simulink model "mw_window"  (R2020a)
settings: Solver=VariableStepAuto  StartTime=0.0  StopTime=inf  RelTol=1e-3
InitFcn:
  | fs = 256e6;
libraries: hdlsllib x6, dspsigops x4, simulink x3
settings Model: Creator=david  LastModifiedBy=david
settings OptimizationCC: BlockReduction=off  ConditionallyExecuteInputs=off  DefaultParameterBehavior=Inlined
settings DebuggingCC: AlgebraicLoopMsg=error
settings HardwareCC: ProdBitPerPointer=32  ProdBitPerSizeT=32  ProdBitPerPtrDiffT=32  ProdLargestAtomicFloat=None  ProdIntDivRoundTo=Undefined  ProdEndianess=Unspecified  ProdWordSize=32  ProdHWDeviceType=ASIC/FPGA->ASIC/FPGA  TargetBitPerPointer=64  TargetBitPerSizeT=64  TargetBitPerPtrDiffT=64  TargetLongLongMode=on  TargetIntDivRoundTo=Zero  TargetEndianess=LittleEndian  TargetWordSize=64  TargetHWDeviceType=Custom Processor->MATLAB Host Computer  ProdEqTarget=off

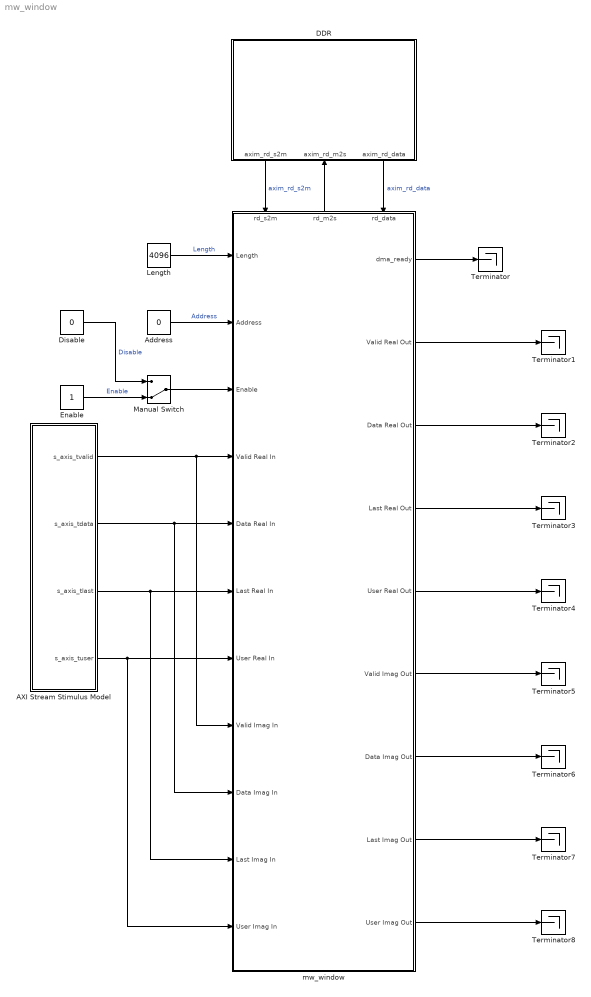
== system mw_window ==
  AXI Stream Stimulus Model : Subsystem
  Address : Constant  Value=0  OutDataTypeStr=uint32  SampleTime=1/fs
  DDR : Subsystem
      settings: PortSchema="{\"entries\":[{\"content\":{\"sides\":[{\"content\":{\"connectorIds\":[]},\"type\":\"ConnectorPlacement.EquallySpacedRectSide\",\"uuid\":\"2b557e1e-8026-43d3-80e6-d6d80e534d60\"},{\"content\":{\"connectorIds\":[\"Out1\",\"In1\",\"Out2\"],\"side\":\"RIGHT\"},\"type\":\"ConnectorPlacement.EquallySpacedRectSide\",\"uuid\":\"d37ff7b5-bcab-46eb-bf2f-7b890d421095\"},{\"content\":{\"connectorIds\":[],\"side\":\"TOP\"},\"type\":\"ConnectorPlacement.EquallySpacedRectSide\",\"uuid\":\"b7392330-958c-44c2-9b9d-e2e6efc00005\"}]},\"type\":\"ConnectorPlacement.EquallySpacedConnector\",\"uuid\":\"d6fedbd7-9a1a-42de-85f8-78943e8230da\"}],\"packageUris\":[\"http://schema.mathworks.com/mf0/Connector/19700101\"],\"version\":\"1.0\"}"
  Disable : Constant  Value=0  OutDataTypeStr=uint32  SampleTime=1/fs
  Enable : Constant  OutDataTypeStr=uint32  SampleTime=1/fs
  Length : Constant  Value=4096  OutDataTypeStr=uint32  SampleTime=1/fs
  Manual Switch : ManualSwitch  CurrentSetting=0
  Terminator{,1..8} (9 alike) : Terminator
  mw_window : Subsystem  TreatAsAtomicUnit=on
      settings: PortSchema="{\"entries\":[{\"content\":{\"sides\":[{\"content\":{\"connectorIds\":[\"In1\",\"In2\",\"In3\",\"In4\",\"In5\",\"In6\",\"In7\",\"In8\",\"In9\",\"In10\",\"In11\"]},\"type\":\"ConnectorPlacement.EquallySpacedRectSide\",\"uuid\":\"9bfde1a4-8e55-439d-ba95-b13ed8c2de82\"},{\"content\":{\"connectorIds\":[\"Out1\",\"Out2\",\"Out3\",\"Out4\",\"Out5\",\"Out6\",\"Out7\",\"Out8\",\"Out9\"],\"side\":\"RIGHT\"},\"type\":\"ConnectorPlacement.EquallySpacedRectSide\",\"uuid\":\"1fa858a7-8a79-448a-a9b9-a47438828a70\"},{\"content\":{\"connectorIds\":[\"In12\",\"Out10\",\"In13\"],\"side\":\"TOP\"},\"type\":\"ConnectorPlacement.EquallySpacedRectSide\",\"uuid\":\"fd991a14-ef2b-4cda-89a6-d580b9713fc0\"}]},\"type\":\"ConnectorPlacement.EquallySpacedConnector\",\"uuid\":\"ee399c2e-0a65-41c3-b55b-7131892126e8\"}],\"packageUris\":[\"http://schema.mathworks.com/mf0/Connector/19700101\"],\"version\":\"1.0\"}"
  wires:
  Length/1 -> mw_window/1(Length)  "Length"
  Address/1 -> mw_window/2(Address)  "Address"
  AXI Stream Stimulus Model/1(s_axis_tvalid) -> mw_window/8(Valid Imag In), mw_window/4(Valid Real In)
  AXI Stream Stimulus Model/2(s_axis_tdata) -> mw_window/9(Data Imag In), mw_window/5(Data Real In)
  AXI Stream Stimulus Model/4(s_axis_tuser) -> mw_window/7(User Real In), mw_window/11(User Imag In)
  AXI Stream Stimulus Model/3(s_axis_tlast) -> mw_window/10(Last Imag In), mw_window/6(Last Real In)
  DDR/2(axim_rd_s2m) -> mw_window/12(rd_s2m)  "axim_rd_s2m"
  mw_window/10(rd_m2s) -> DDR/1(axim_rd_m2s)
  DDR/1(axim_rd_data) -> mw_window/13(rd_data)  "axim_rd_data"
  mw_window/1(dma_ready) -> Terminator/1
  mw_window/2(Valid Real Out) -> Terminator1/1
  mw_window/3(Data Real Out) -> Terminator2/1
  mw_window/4(Last Real Out) -> Terminator3/1
  mw_window/5(User Real Out) -> Terminator4/1
  mw_window/6(Valid Imag Out) -> Terminator5/1
  mw_window/7(Data Imag Out) -> Terminator6/1
  mw_window/8(Last Imag Out) -> Terminator7/1
  mw_window/9(User Imag Out) -> Terminator8/1
  Manual Switch/1 -> mw_window/3(Enable)
  Disable/1 -> Manual Switch/1  "Disable"
  Enable/1 -> Manual Switch/2  "Enable"

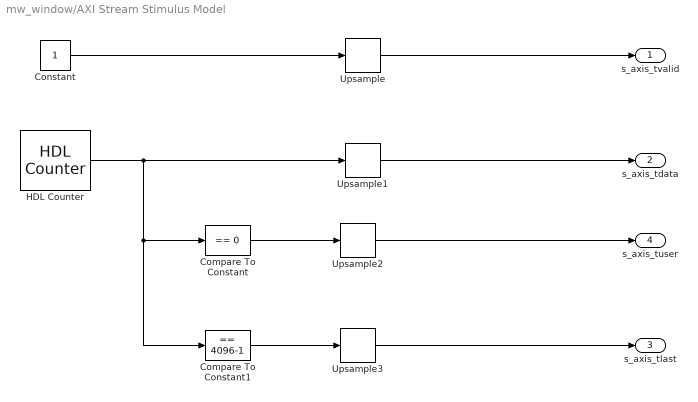
== system mw_window/AXI Stream Stimulus Model ==
  Compare To Constant : simulink/Logic and Bit Operations/Compare To Constant  relop===  const=0  OutDataTypeStr=boolean
  Compare To Constant1 : simulink/Logic and Bit Operations/Compare To Constant  relop===  const=4096-1  OutDataTypeStr=boolean
  Constant : Constant  OutDataTypeStr=boolean  SampleTime=-1
  HDL Counter : hdlsllib/Sources/HDL Counter  CountType=Count limited  CountInit=0  CountStep=1  CountMax=4096-1  CountFromType=Initial value  CountFrom=0  CountResetPort=off  CountLoadPort=off  CountEnbPort=off  CountDirPort=off  CountDataType=Unsigned  CountWordLen=16  CountFracLen=0  CountSampTime=-1
  Upsample{,1..3} (4 alike) : dspsigops/Upsample  N=2  phase=0  RateOptions=Allow multirate processing  ic=0  mode=Unused parameter value
  s_axis_tvalid : Outport
  s_axis_tdata : Outport  Port=2
  s_axis_tlast : Outport  Port=3
  s_axis_tuser : Outport  Port=4
  wires:
  Constant/1 -> Upsample/1
  Compare To Constant/1 -> Upsample2/1
  Compare To Constant1/1 -> Upsample3/1
  HDL Counter/1 -> Upsample1/1, Compare To Constant1/1, Compare To Constant/1
  Upsample/1 -> s_axis_tvalid/1
  Upsample1/1 -> s_axis_tdata/1
  Upsample2/1 -> s_axis_tuser/1
  Upsample3/1 -> s_axis_tlast/1

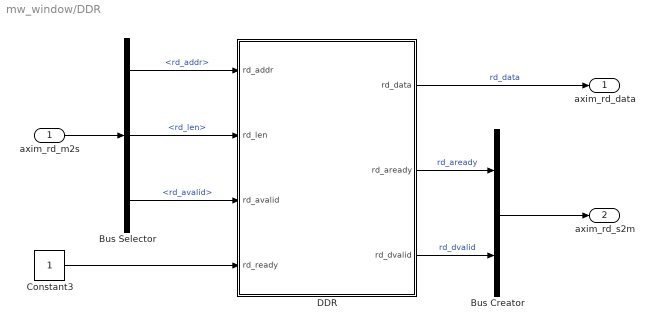
== system mw_window/DDR ==
  axim_rd_m2s : Inport
  Bus Creator : BusCreator  Inputs=2
  Bus Selector : BusSelector  OutputSignals=rd_addr,rd_len,rd_avalid
  Constant3 : Constant  OutDataTypeStr=boolean  SampleTime=-1
  DDR : Subsystem  mask{DDR_DATA=uint16(ones(1,4096)*2^15)}
      mask init:
      | %load('ram_data');
  axim_rd_data : Outport  VectorParamsAs1DForOutWhenUnconnected=off
  axim_rd_s2m : Outport  Port=2  VectorParamsAs1DForOutWhenUnconnected=off
  wires:
  Bus Creator/1 -> axim_rd_s2m/1
  DDR/1(rd_data) -> axim_rd_data/1  "rd_data"
  DDR/3(rd_dvalid) -> Bus Creator/2  "rd_dvalid"
  Constant3/1 -> DDR/4(rd_ready)
  Bus Selector/1 -> DDR/1(rd_addr)  "<rd_addr>"
  axim_rd_m2s/1 -> Bus Selector/1
  Bus Selector/3 -> DDR/3(rd_avalid)  "<rd_avalid>"
  DDR/2(rd_aready) -> Bus Creator/1  "rd_aready"
  Bus Selector/2 -> DDR/2(rd_len)  "<rd_len>"

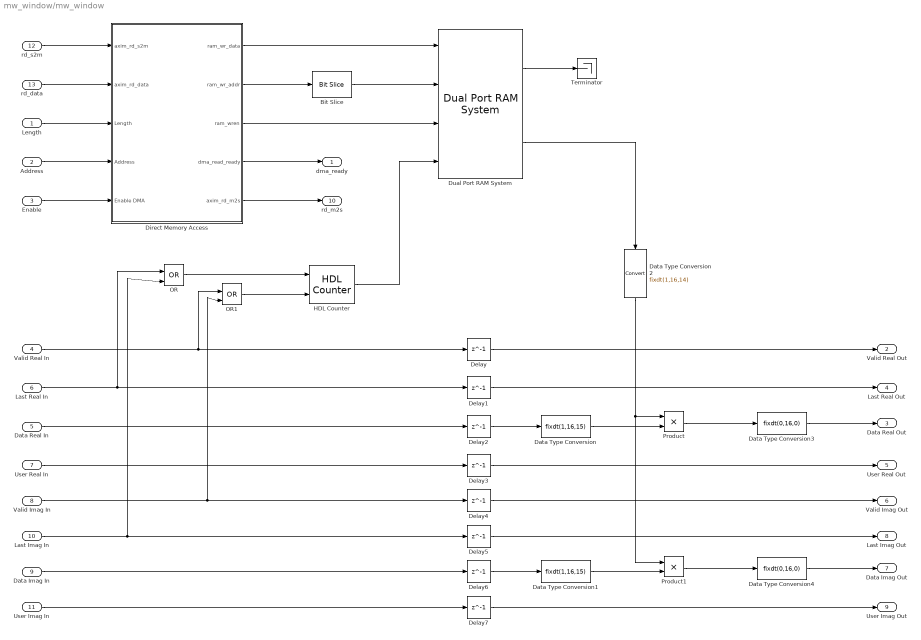
== system mw_window/mw_window ==
  Length : Inport
  Address : Inport  Port=2
  Enable : Inport  Port=3
  Valid Real In : Inport  Port=4
  Data Real In : Inport  Port=5
  Last Real In : Inport  Port=6
  User Real In : Inport  Port=7
  Valid Imag In : Inport  Port=8
  Data Imag In : Inport  Port=9
  Last Imag In : Inport  Port=10
  User Imag In : Inport  Port=11
  rd_s2m : Inport  Port=12
  rd_data : Inport  Port=13
  Bit Slice : hdlsllib/Logic and Bit Operations/Bit Slice  lidx=12  ridx=0
      settings: SourceProductBaseCode=SL
  Data Type Conversion : DataTypeConversion  OutDataTypeStr=fixdt(1,16,15)  ConvertRealWorld=Stored Integer (SI)
  Data Type Conversion1 : DataTypeConversion  OutDataTypeStr=fixdt(1,16,15)  ConvertRealWorld=Stored Integer (SI)
  Data Type Conversion2 : DataTypeConversion  OutDataTypeStr=fixdt(1,16,14)  ConvertRealWorld=Stored Integer (SI)
  Data Type Conversion3 : DataTypeConversion  OutDataTypeStr=fixdt(0,16,0)  ConvertRealWorld=Stored Integer (SI)
  Data Type Conversion4 : DataTypeConversion  OutDataTypeStr=fixdt(0,16,0)  ConvertRealWorld=Stored Integer (SI)
  Delay{,1..7} (8 alike) : Delay  DelayLength=1
  Direct Memory Access : Subsystem
  Dual Port RAM System : hdlsllib/HDL RAMs/Dual Port RAM System  RAMType=Dual port  WriteOutputValue=New data  RAMInitialValue=ones(1, 2^13)*2^14  SimulateUsing=Code generation
      settings: SourceProductBaseCode=SL
  HDL Counter : hdlsllib/Sources/HDL Counter  CountType=Count limited  CountInit=0  CountStep=1  CountMax=4095  CountFromType=Initial value  CountFrom=0  CountResetPort=on  CountLoadPort=off  CountEnbPort=on  CountDirPort=off  CountDataType=Unsigned  CountWordLen=13  CountFracLen=0  CountSampTime=1
  OR : Logic  Operator=OR  IconShape=distinctive  AllPortsSameDT=off  OutDataTypeStr=boolean
  OR1 : Logic  Operator=OR  IconShape=distinctive  AllPortsSameDT=off  OutDataTypeStr=boolean
  Product : Product  OutDataTypeStr=fixdt(1,16,15)  RndMeth=Round  SaturateOnIntegerOverflow=on
  Product1 : Product  OutDataTypeStr=fixdt(1,16,15)  RndMeth=Round  SaturateOnIntegerOverflow=on
  Terminator : Terminator
  dma_ready : Outport
  Valid Real Out : Outport  Port=2
  Data Real Out : Outport  Port=3
  Last Real Out : Outport  Port=4
  User Real Out : Outport  Port=5
  Valid Imag Out : Outport  Port=6
  Data Imag Out : Outport  Port=7
  Last Imag Out : Outport  Port=8
  User Imag Out : Outport  Port=9
  rd_m2s : Outport  Port=10
  wires:
  Address/1 -> Direct Memory Access/4(Address)
  Enable/1 -> Direct Memory Access/5(Enable DMA)
  Length/1 -> Direct Memory Access/3(Length)
  Direct Memory Access/1(ram_wr_data) -> Dual Port RAM System/1
  Direct Memory Access/2(ram_wr_addr) -> Bit Slice/1
  Direct Memory Access/3(ram_wren) -> Dual Port RAM System/3
  Direct Memory Access/4(dma_read_ready) -> dma_ready/1
  HDL Counter/1 -> Dual Port RAM System/4
  Valid Real In/1 -> OR1/1, Delay/1
  Last Real In/1 -> OR/1, Delay1/1
  Dual Port RAM System/1 -> Terminator/1
  Direct Memory Access/5(axim_rd_m2s) -> rd_m2s/1
  Dual Port RAM System/2 -> Data Type Conversion2/1
  Data Real In/1 -> Delay2/1
  Product/1 -> Data Type Conversion3/1
  User Real In/1 -> Delay3/1
  OR/1 -> HDL Counter/1
  OR1/1 -> HDL Counter/2
  Last Imag In/1 -> OR/2, Delay5/1
  Valid Imag In/1 -> OR1/2, Delay4/1
  Data Imag In/1 -> Delay6/1
  Product1/1 -> Data Type Conversion4/1
  User Imag In/1 -> Delay7/1
  rd_s2m/1 -> Direct Memory Access/1(axim_rd_s2m)
  rd_data/1 -> Direct Memory Access/2(axim_rd_data)
  Data Type Conversion/1 -> Product/2
  Data Type Conversion1/1 -> Product1/2
  Data Type Conversion2/1 -> Product1/1, Product/1
  Data Type Conversion3/1 -> Data Real Out/1
  Data Type Conversion4/1 -> Data Imag Out/1
  Delay/1 -> Valid Real Out/1
  Delay1/1 -> Last Real Out/1
  Delay2/1 -> Data Type Conversion/1
  Delay3/1 -> User Real Out/1
  Delay4/1 -> Valid Imag Out/1
  Delay5/1 -> Last Imag Out/1
  Delay6/1 -> Data Type Conversion1/1
  Delay7/1 -> User Imag Out/1
  Bit Slice/1 -> Dual Port RAM System/2

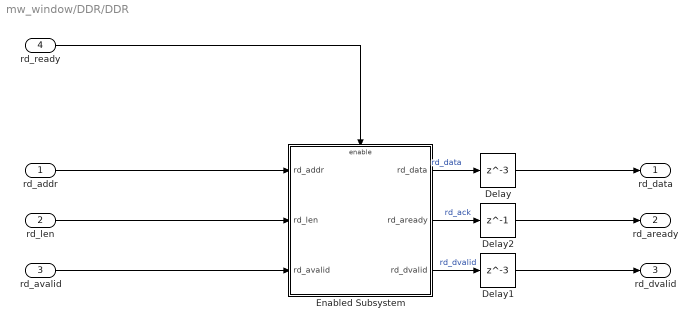
== system mw_window/DDR/DDR ==
  rd_addr : Inport
  rd_len : Inport  Port=2
  rd_avalid : Inport  Port=3
  rd_ready : Inport  Port=4
  Delay : Delay  DelayLength=3
  Delay1 : Delay  DelayLength=3
  Delay2 : Delay  DelayLength=1
  Enabled Subsystem : Subsystem  TreatAsAtomicUnit=on
  rd_data : Outport  VectorParamsAs1DForOutWhenUnconnected=off
  rd_aready : Outport  Port=2  VectorParamsAs1DForOutWhenUnconnected=off
  rd_dvalid : Outport  Port=3  VectorParamsAs1DForOutWhenUnconnected=off
  wires:
  Delay2/1 -> rd_aready/1
  Delay1/1 -> rd_dvalid/1
  Enabled Subsystem/3(rd_dvalid) -> Delay1/1  "rd_dvalid"
  rd_ready/1 -> Enabled Subsystem/Enable
  Enabled Subsystem/2(rd_aready) -> Delay2/1  "rd_ack"
  rd_avalid/1 -> Enabled Subsystem/3(rd_avalid)
  Delay/1 -> rd_data/1
  Enabled Subsystem/1(rd_data) -> Delay/1  "rd_data"
  rd_len/1 -> Enabled Subsystem/2(rd_len)
  rd_addr/1 -> Enabled Subsystem/1(rd_addr)

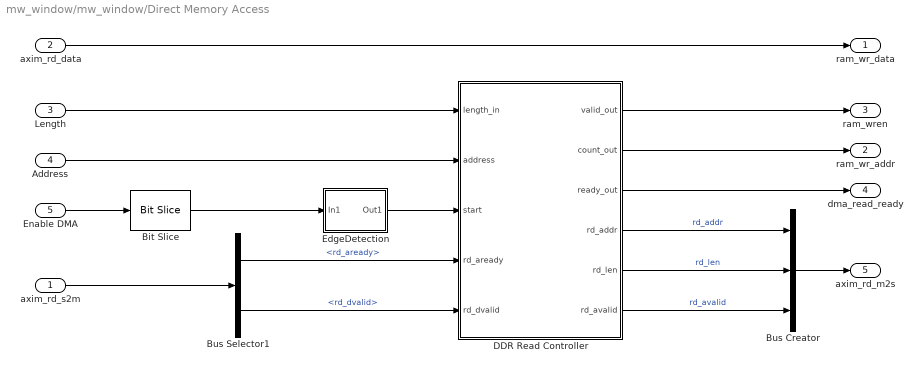
== system mw_window/mw_window/Direct Memory Access ==
  axim_rd_s2m : Inport
  axim_rd_data : Inport  Port=2
  Length : Inport  Port=3
  Address : Inport  Port=4
  Enable DMA : Inport  Port=5
  Bit Slice : hdlsllib/Logic and Bit Operations/Bit Slice  lidx=0  ridx=0
      settings: SourceProductBaseCode=SL
  Bus Creator : BusCreator  Inputs=3
  Bus Selector1 : BusSelector  OutputSignals=rd_aready,rd_dvalid
  DDR Read Controller : MATLAB Function  TreatAsAtomicUnit=on
  EdgeDetection : Subsystem
  ram_wr_data : Outport  VectorParamsAs1DForOutWhenUnconnected=off
  ram_wr_addr : Outport  Port=2  VectorParamsAs1DForOutWhenUnconnected=off
  ram_wren : Outport  Port=3  VectorParamsAs1DForOutWhenUnconnected=off
  dma_read_ready : Outport  Port=4  VectorParamsAs1DForOutWhenUnconnected=off
  axim_rd_m2s : Outport  Port=5  VectorParamsAs1DForOutWhenUnconnected=off
  wires:
  Enable DMA/1 -> Bit Slice/1
  Address/1 -> DDR Read Controller/2(address)
  DDR Read Controller/4(rd_addr) -> Bus Creator/1  "rd_addr"
  DDR Read Controller/6(rd_avalid) -> Bus Creator/3  "rd_avalid"
  Bus Creator/1 -> axim_rd_m2s/1
  DDR Read Controller/5(rd_len) -> Bus Creator/2  "rd_len"
  Bus Selector1/1 -> DDR Read Controller/4(rd_aready)  "<rd_aready>"
  axim_rd_s2m/1 -> Bus Selector1/1
  Bus Selector1/2 -> DDR Read Controller/5(rd_dvalid)  "<rd_dvalid>"
  axim_rd_data/1 -> ram_wr_data/1
  DDR Read Controller/2(count_out) -> ram_wr_addr/1
  DDR Read Controller/1(valid_out) -> ram_wren/1
  EdgeDetection/1(Out1) -> DDR Read Controller/3(start)
  DDR Read Controller/3(ready_out) -> dma_read_ready/1
  Length/1 -> DDR Read Controller/1(length_in)
  Bit Slice/1 -> EdgeDetection/1(In1)

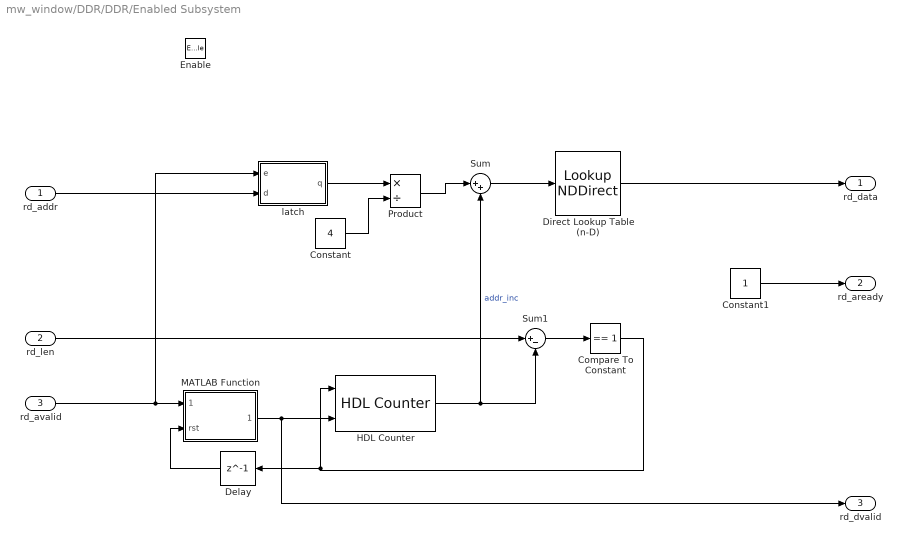
== system mw_window/DDR/DDR/Enabled Subsystem ==
  rd_addr : Inport
  rd_len : Inport  Port=2
  rd_avalid : Inport  Port=3
  Enable : EnablePort
  Compare To Constant : simulink/Logic and Bit Operations/Compare To Constant  relop===  const=1  OutDataTypeStr=boolean
  Constant : Constant  Value=4  SampleTime=-1
  Constant1 : Constant  OutDataTypeStr=boolean  SampleTime=-1
  Delay : Delay  DelayLength=1
  Direct Lookup Table (n-D) : LookupNDDirect  NumberOfTableDimensions=1  Table=DDR_DATA  DiagnosticForOutOfRangeInput=Error
  HDL Counter : hdlsllib/Sources/HDL Counter  CountType=Count limited  CountInit=0  CountStep=1  CountMax=2^16-1  CountFromType=Specify  CountFrom=0  CountResetPort=on  CountLoadPort=off  CountEnbPort=on  CountDirPort=off  CountDataType=Unsigned  CountWordLen=16  CountFracLen=0  CountSampTime=1
  MATLAB Function : MATLAB Function  TreatAsAtomicUnit=on
  Product : Product  Inputs=*/
  Sum : Sum  Inputs=|++  OutDataTypeStr=uint32
  Sum1 : Sum  Inputs=|+-
  latch : Subsystem
  rd_data : Outport  VectorParamsAs1DForOutWhenUnconnected=off
  rd_aready : Outport  Port=2  VectorParamsAs1DForOutWhenUnconnected=off
  rd_dvalid : Outport  Port=3  VectorParamsAs1DForOutWhenUnconnected=off
  wires:
  Constant1/1 -> rd_aready/1
  Delay/1 -> MATLAB Function/2(rst)
  Constant/1 -> Product/2
  Product/1 -> Sum/1
  latch/1(q) -> Product/1
  MATLAB Function/1(start_counter) -> HDL Counter/2, rd_dvalid/1
  rd_avalid/1 -> MATLAB Function/1(rd_avalid), latch/1(e)
  rd_len/1 -> Sum1/1
  rd_addr/1 -> latch/2(d)
  Compare To Constant/1 -> HDL Counter/1, Delay/1
  Sum/1 -> Direct Lookup Table (n-D)/1
  Sum1/1 -> Compare To Constant/1
  HDL Counter/1 -> Sum/2, Sum1/2  "addr_inc"
  Direct Lookup Table (n-D)/1 -> rd_data/1

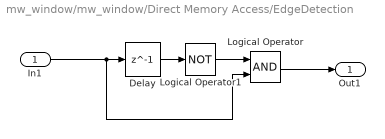
== system mw_window/mw_window/Direct Memory Access/EdgeDetection ==
  In1 : Inport
  Delay : Delay  DelayLength=1
  Logical Operator : Logic  AllPortsSameDT=off  OutDataTypeStr=boolean
  Logical Operator1 : Logic  Operator=NOT  AllPortsSameDT=off  OutDataTypeStr=boolean
  Out1 : Outport  VectorParamsAs1DForOutWhenUnconnected=off
  wires:
  Logical Operator/1 -> Out1/1
  Logical Operator1/1 -> Logical Operator/1
  Delay/1 -> Logical Operator1/1
  In1/1 -> Delay/1, Logical Operator/2

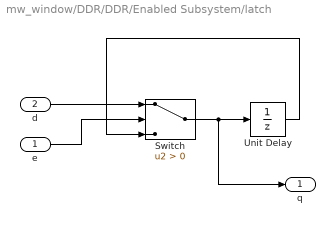
== system mw_window/DDR/DDR/Enabled Subsystem/latch ==
  e : Inport  OutDataTypeStr=boolean
  d : Inport  Port=2
  Switch : Switch  Criteria=u2 > Threshold
  Unit Delay : UnitDelay  SampleTime=-1  HasFrameUpgradeWarning=on
  q : Outport  VectorParamsAs1DForOutWhenUnconnected=off
  wires:
  Switch/1 -> Unit Delay/1, q/1
  e/1 -> Switch/2
  Unit Delay/1 -> Switch/3
  d/1 -> Switch/1

== matlab function mw_window/DDR/DDR/Enabled Subsystem/MATLAB Function ==
  data: rd_avalid input; start_counter output; rst input
function start_counter  = fcn(rd_avalid, rst)

persistent start;
if(isempty(start))
    start = false;
end

if (rd_avalid == true)
    start = true;
else
    
    if (rst == true)
        start = false;
    else
        start = start;
    end
end
start_counter = start;

== matlab function mw_window/Direct Memory Access/DDR Read Controller ==
  data: valid_out output boolean; count_out output; ready_out output boolean; length_in input; address input; start input boolean; rd_aready input; rd_dvalid input; rd_addr output uint32; rd_len output; rd_avalid output
function [valid_out,count_out,ready_out,rd_addr,rd_len,rd_avalid] = ddr_read_control(length_in, address, start, rd_aready, rd_dvalid)

% Create persistent variables (registers)
persistent burst_stop
if(isempty(burst_stop))
    burst_stop = uint16(0);
end
persistent burst_count;
if(isempty(burst_count))
    burst_count = uint16(0);
end
persistent rstate;
if isempty(rstate)
    rstate = fi(0, 0, 4, 0);
end


% State Memory Encoding
IDLE             = fi(1, 0, 4, 0);
READ_BURST_START = fi(2, 0, 4, 0);
DATA_COUNT       = fi(4, 0, 4, 0);

% Read control state machine
switch (rstate)
    case IDLE
        % output to AXI4 Master
        rd_addr = address;
        rd_len = uint16(0);
        rd_avalid = false;
        
        % output to DUT
        valid_out = false;
        ready_out = true;
        count_out = uint16(0);
        
        % State vars
        burst_count = uint16(0);
        burst_stop = uint16(length_in);
        
        if rd_aready && start
            rstate(:) = READ_BURST_START;
        end
        
    case READ_BURST_START
        % output to AXI4 Master
        rd_addr = address;
        rd_len = uint16(burst_stop);
        rd_avalid = true;
        
        % output to DUT
        valid_out = false;
        count_out = uint16(0);
        ready_out = false;
        
        rstate(:) = DATA_COUNT;
        
    case DATA_COUNT
        % output to AXI4 Master
        rd_addr = address;
        rd_len = uint16(burst_stop);
        rd_avalid = false;
        
        % output to DUT
        valid_out = rd_dvalid;
        count_out = uint16(burst_count);
        ready_out = false;
        
        % State vars
        if ( rd_dvalid )
            burst_count = uint16(burst_count + 1);
        end
        
        if ( burst_count == burst_stop )
            rstate(:) = IDLE;
        else
            rstate(:) = DATA_COUNT;
        end
        
    otherwise
        % output to AXI4 Master
        rd_addr = uint32(0);
        rd_len = uint16(0);
        rd_avalid = false;
        
        % output to DUT
        valid_out = false;
        count_out = uint16(0);
        ready_out = false;
        
        rstate(:) = IDLE;
end

end
